simulink model "WaveSimulator"  (R2019a)
settings: Solver=FixedStepAuto  StartTime=0.0  StopTime=240  FixedStep=0.005  RelTol=1e-3
undefined symbols (not defined in the file or in its folder): lambda, PolePlacer, sigma, w0
libraries: simulink x3, aerolibconvert2 x1, cstblocks x1
settings Model: Creator=motionlab  LastModifiedBy=motionlab
settings DataIOCC: ReturnWorkspaceOutputs=off
settings OptimizationCC: LocalBlockOutputs=off
settings DebuggingCC: ArithmeticOperatorsInVariantConditions=warning
settings SFSimCC: SimUseLocalCustomCode=off
settings RTWCC: SystemTargetFile=TwinCAT.tlc  GenCodeOnly=on  MakeCommand=make_tct  TemplateMakefile=tct_msbuild.tmf  Description=TwinCAT Target  GenerateReport=on  RTWUseLocalCustomCode=off  TargetLang=C++
settings STFCustomTargetCC: TargetLangStandard=C++03 (ISO)  CompOptLevelCompliant=on  MATLABClassNameForMDSCustomization=Simulink.SoftwareTarget.TargetSpecificTriggerConfigurationBase  SystemTargetFile=TwinCAT.tlc

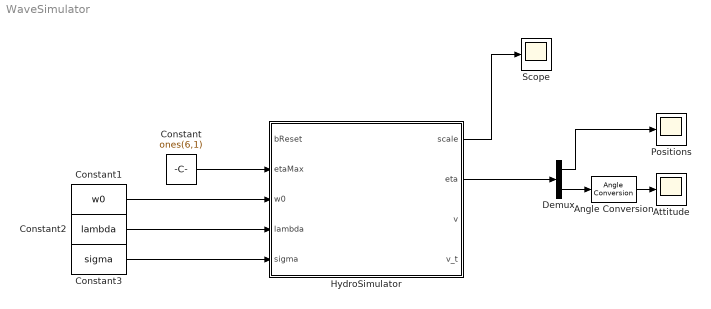
== system WaveSimulator ==
  Angle Conversion : aerolibconvert2/Angle Conversion  IU=rad  OU=deg
  Attitude : Scope
  Constant : Constant  Value=ones(6,1)
  Constant1 : Constant  Value=w0
  Constant2 : Constant  Value=lambda
  Constant3 : Constant  Value=sigma
  Demux : Demux  Outputs=2
  HydroSimulator : Subsystem
  Positions : Scope
  Scope : Scope
  wires:
  Angle Conversion/1 -> Attitude/1
  Demux/1 -> Positions/1
  Demux/2 -> Angle Conversion/1
  HydroSimulator/2(eta) -> Demux/1
  Constant/1 -> HydroSimulator/2(etaMax)
  Constant1/1 -> HydroSimulator/3(w0)
  Constant2/1 -> HydroSimulator/4(lambda)
  Constant3/1 -> HydroSimulator/5(sigma)
  HydroSimulator/1(scale) -> Scope/1

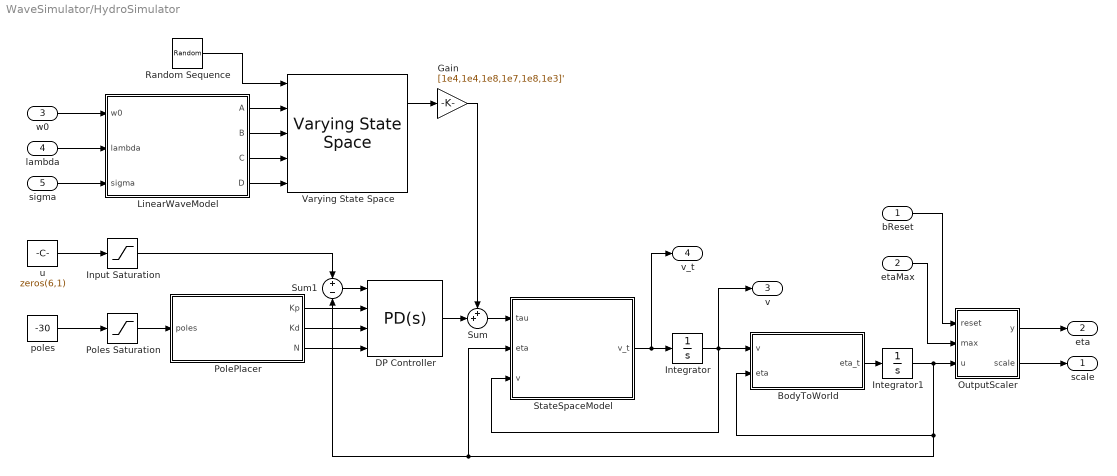
== system WaveSimulator/HydroSimulator ==
  bReset : Inport  OutDataTypeStr=boolean  PortDimensions=1
  etaMax : Inport  Port=2  PortDimensions=6
  w0 : Inport  Port=3
  lambda : Inport  Port=4
  sigma : Inport  Port=5
  BodyToWorld : MATLAB Function  TreatAsAtomicUnit=on
  DP Controller : simulink/Continuous/PID Controller  Controller=PD  Form=Parallel  TimeDomain=Continuous-time  SampleTime=-1  IntegratorMethod=Forward Euler  FilterMethod=Forward Euler  ControllerParametersSource=external  P=PolePlacer(3, 100, 'P')  I=1  D=PolePlacer(3, 100, 'D')  UseFilter=on  N=100  TunerSelectOption=Transfer Function Based (PID Tuner App)  InitialConditionSource=internal  InitialConditionForIntegrator=0  InitialConditionForFilter=0  DifferentiatorICPrevScaledInput=0  ExternalReset=none  TrackingMode=off  Kt=1  LimitOutput=off  UpperSaturationLimit=inf  LowerSaturationLimit=-inf  LinearizeAsGain=on  AntiWindupMode=none  Kb=1  POutMin=[]  POutMax=[]  IOutMin=[]  IOutMax=[]  DOutMin=[]  DOutMax=[]  NOutMin=[]  NOutMax=[]  SumOutMin=[]  SumOutMax=[]  SaturationOutMin=[]  SaturationOutMax=[]  PParamMin=[]  PParamMax=[]  IParamMin=[]  IParamMax=[]  DParamMin=[]  DParamMax=[]  NParamMin=[]  NParamMax=[]  KbParamMin=[]  KbParamMax=[]  KtParamMin=[]  KtParamMax=[]  KbOutMin=[]  KbOutMax=[]  KtOutMin=[]  KtOutMax=[]  IntegratorOutMin=[]  IntegratorOutMax=[]  FilterOutMin=[]  FilterOutMax=[]  SumI1OutMin=[]  SumI1OutMax=[]  SumI2OutMin=[]  SumI2OutMax=[]  SumI3OutMin=[]  SumI3OutMax=[]  SumI4OutMin=[]  SumI4OutMax=[]  SumDOutMin=[]  SumDOutMax=[]  DifferentiatorOutMin=[]  DifferentiatorOutMax=[]  FilterDiffOutCoefMin=[]  FilterDiffOutCoefMax=[]  ReciprocalOutMin=[]  ReciprocalOutMax=[]  SumDenOutMin=[]  SumDenOutMax=[]  SumNumOutMin=[]  SumNumOutMax=[]  DivideOutMin=[]  DivideOutMax=[]  IntegratorContinuousStateAttributes=''  IntegratorStateMustResolveToSignalObject=off  IntegratorRTWStateStorageClass=Auto  FilterContinuousStateAttributes=''  FilterStateMustResolveToSignalObject=off  FilterRTWStateStorageClass=Auto  ParallelPVariant=ExternalParameters  IdealPVariant=Disabled  IVariant=Disabled  DVariant=ExternalParameters  IntegratorVariant=Disabled  SatVariant=Disabled  AWVariant=Disabled  PCopyVariant=Disabled  TRVariant=Disabled  FdbkBlocksVariant=Forward  IdealPFdbkVariant=Disabled  SatFdbkVariant=Disabled  DerivativeFilterVariant=ContFilter  NVariant=ExternalParameters  NCopyVariant=Disabled  FilterICVariant=InternalICsFilter  IntegratorICVariant=Disabled  ExternalResetVariant=Disabled  TRSumVariant=Passthrough  SumFdbkVariant=Disabled  SumVariant=Sum_PD
  Gain : Gain  Gain=[1e4,1e4,1e8,1e7,1e8,1e3]'
  Input Saturation : Saturate  UpperLimit=[0.2, 0.2, 0, 0, 0, 5/180*pi]  LowerLimit=-[0.2, 0.2, 0, 0, 0, 5/180*pi]
  Integrator : Integrator  InitialCondition=zeros(6,1)
  Integrator1 : Integrator  InitialCondition=zeros(6,1)
  LinearWaveModel : MATLAB Function  TreatAsAtomicUnit=on  SystemSampleTime=1
  OutputScaler : Subsystem
  PolePlacer : MATLAB Function  TreatAsAtomicUnit=on  SystemSampleTime=1
  Poles Saturation : Saturate  UpperLimit=0  LowerLimit=-30
  Random Sequence : RandomNumber  Mean=zeros(6,1)  Variance=ones(6,1)  Seed=[0,20,500,9000,400,200]  SampleTime=0.01
  StateSpaceModel : MATLAB Function  TreatAsAtomicUnit=on
  Sum : Sum  Inputs=++|
  Sum1 : Sum  Inputs=+|-
  Varying State Space : cstblocks/Linear Parameter Varying/Varying State Space  x0=zeros(12,1)'  xNames=''  OutputX=on  OutputDX=off
      settings: SourceProductName=Control System Toolbox
  poles : Constant  Value=-30
  u : Constant  Value=zeros(6,1)
  scale : Outport
  eta : Outport  Port=2
  v : Outport  Port=3
  v_t : Outport  Port=4
  wires:
  Random Sequence/1 -> Varying State Space/1
  DP Controller/1 -> Sum/2
  StateSpaceModel/1(v_t) -> v_t/1, Integrator/1
  BodyToWorld/1(eta_t) -> Integrator1/1
  Sum1/1 -> DP Controller/1
  Sum/1 -> StateSpaceModel/1(tau)
  Integrator/1 -> v/1, BodyToWorld/1(v), StateSpaceModel/3(v)
  PolePlacer/2(Kd) -> DP Controller/3
  PolePlacer/3(N) -> DP Controller/4
  PolePlacer/1(Kp) -> DP Controller/2
  LinearWaveModel/1(A) -> Varying State Space/2
  LinearWaveModel/3(C) -> Varying State Space/4
  LinearWaveModel/2(B) -> Varying State Space/3
  LinearWaveModel/4(D) -> Varying State Space/5
  Varying State Space/1 -> Gain/1
  Gain/1 -> Sum/1
  u/1 -> Input Saturation/1
  Poles Saturation/1 -> PolePlacer/1(poles)
  poles/1 -> Poles Saturation/1
  Input Saturation/1 -> Sum1/1
  Integrator1/1 -> OutputScaler/3(u), Sum1/2, StateSpaceModel/2(eta), BodyToWorld/2(eta)
  bReset/1 -> OutputScaler/1(reset)
  etaMax/1 -> OutputScaler/2(max)
  OutputScaler/1(y) -> eta/1
  OutputScaler/2(scale) -> scale/1
  w0/1 -> LinearWaveModel/1(w0)
  lambda/1 -> LinearWaveModel/2(lambda)
  sigma/1 -> LinearWaveModel/3(sigma)

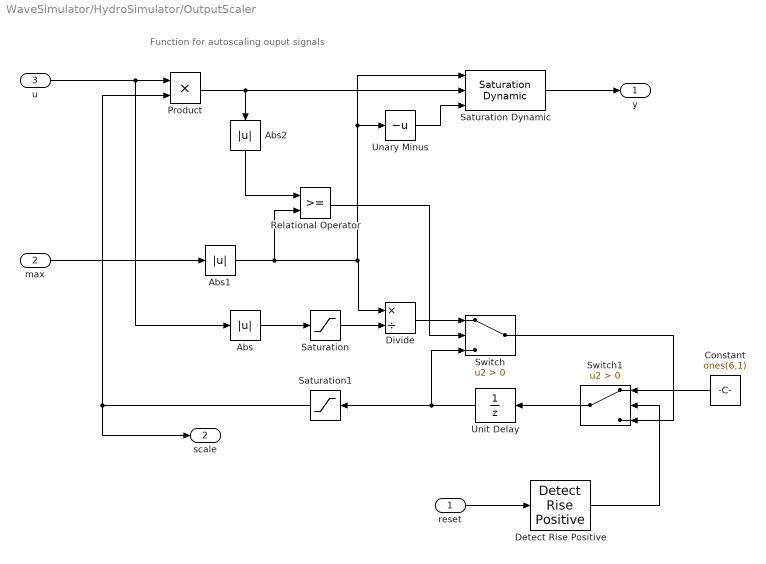
== system WaveSimulator/HydroSimulator/OutputScaler ==
  note: Function for autoscaling ouput signals
  reset : Inport  OutDataTypeStr=boolean
  max : Inport  Port=2
  u : Inport  Port=3
  Abs : Abs
  Abs1 : Abs
  Abs2 : Abs
  Constant : Constant  Value=ones(6,1)
  Detect Rise Positive : simulink/Logic and Bit Operations/Detect Rise Positive  vinit=0  OutDataTypeStr=boolean
  Divide : Product  Inputs=*/
  Product : Product
  Relational Operator : RelationalOperator  OutDataTypeStr=boolean  RndMeth=Nearest
  Saturation : Saturate  UpperLimit=inf  LowerLimit=1e-6
  Saturation Dynamic : simulink/Discontinuities/Saturation Dynamic  OutMin=[]  OutMax=[]  OutDataTypeStr=Inherit: Same as second input  OutDataType=fixdt(1, 16)  OutScaling=2^-10  DoSatur=off
  Saturation1 : Saturate  UpperLimit=1  LowerLimit=1e-10
  Switch : Switch  Criteria=u2 > Threshold
  Switch1 : Switch  Criteria=u2 > Threshold
  Unary Minus : UnaryMinus
  Unit Delay : UnitDelay  InitialCondition=1  SampleTime=-1  HasFrameUpgradeWarning=on
  y : Outport
  scale : Outport  Port=2
  wires:
  Relational Operator/1 -> Switch/2
  Unit Delay/1 -> Saturation1/1, Switch/3
  Abs1/1 -> Relational Operator/2, Unary Minus/1, Saturation Dynamic/1, Divide/1
  Divide/1 -> Switch/1
  Saturation/1 -> Divide/2
  Abs/1 -> Saturation/1
  u/1 -> Product/1, Abs/1
  Unary Minus/1 -> Saturation Dynamic/3
  Product/1 -> Saturation Dynamic/2, Abs2/1
  Abs2/1 -> Relational Operator/1
  Saturation1/1 -> Product/2, scale/1
  Saturation Dynamic/1 -> y/1
  max/1 -> Abs1/1
  reset/1 -> Detect Rise Positive/1
  Switch1/1 -> Unit Delay/1
  Detect Rise Positive/1 -> Switch1/2
  Switch/1 -> Switch1/3
  Constant/1 -> Switch1/1

== matlab function WaveSimulator/HydroSimulator/BodyToWorld ==
  data: v input; eta_t output; eta input
function eta_t  = BodyToWorld(v, eta)

% Vessel kinemamtics
phi = eta(4:6);

J = eye(6);

% Fossen's hydrodynamics jacobian version
J(1:3,1:3) = math3d.Rz(phi(3))*math3d.Ry(phi(2))*math3d.Rx(phi(1));
J(4:6,4:6) = math3d.Tphi(phi, 'zyx');

% {b} -> {n}
eta_t = J*v;
    
end

== matlab function WaveSimulator/HydroSimulator/StateSpaceModel ==
  data: tau input; eta input; v_t output; v input
function v_t = StateSpaceModel(tau, eta, v)

    % Load data from mss file
    data = coder.load('supply.mat');

    v_t = zeros(6,1);
    
    v_t = data.supply.Minv*(tau - data.supply.D*v - data.supply.G*eta);

end

== matlab function WaveSimulator/HydroSimulator/PolePlacer ==
  data: poles input; Kp output; Kd output; N output
function [Kp, Kd, N] = PolePlacer(poles)
    
    % Load estimated 1st order model data for surge, sway and yaw motion
    data = coder.load('step.mat');
    
    % 1st order plant paramaters
    Kss = [
            data.step.surge.Kss,
            data.step.sway.Kss,
            data.step.yaw.Kss
        ];
    
    tau = [
            data.step.surge.tau,
            data.step.sway.tau,
            data.step.yaw.tau
        ];
    
    Kp = zeros(6,1);
    Kd = zeros(6,1);
    
    % Calculate gains analytically 
    N = 100;
    
    poles = abs(poles);
    
    Kp(1) = (tau(1)*poles^2 - N)/(Kss(1)*N);
    Kp(2) = (tau(2)*poles^2 - N)/(Kss(2)*N);
    Kp(6) = (tau(3)*poles^2 - N)/(Kss(3)*N);
    
    Kd(1) = (2*tau(1)*poles - 1 - Kp(1)*Kss(1) - tau(1)*N)/(Kss(1)*N);
    Kd(2) = (2*tau(2)*poles - 1 - Kp(2)*Kss(2) - tau(2)*N)/(Kss(2)*N);
    Kd(6) = (2*tau(3)*poles - 1 - Kp(6)*Kss(3) - tau(3)*N)/(Kss(3)*N);
    
    Kp = abs(Kp);
    Kd = abs(Kd);
end

== matlab function WaveSimulator/HydroSimulator/LinearWaveModel ==
  data: w0 input; A output; B output; C output; lambda input; sigma input; D output
function [A, B, C, D] = LinearWaveModel(w0, lambda, sigma)
    
    % p. 216-220 in "Fossen, T. I. (2011). Handbook of Marine Craft
    % Hydrodynamics and Motion Control"
    
    
    % Linearized wave spectrum model matrices
    
    Kw = abs(2*lambda*w0*sigma);
    
    % A
    a = [    0,                 1;
         -w0^2, -2*abs(lambda*w0)];
    
    A = blkdiag(a,a,a,a,a,a);
    
    % B
    b = [0; Kw];
    
    B = blkdiag(b,b,b,b,b,b);
    
    % C
    c = [0, 1];
    
    C = blkdiag(c,c,c,c,c,c);
    
    % D
    D = zeros(6,6);
    
end
